simulink model "FIR_Input160M_Output200M"  (R2023b)
settings: Solver=ode45  StartTime=0.0  StopTime=100000/200e6  RelTol=1e-3  EnableMultiTasking=on
undefined symbols (not defined in the file): xc7vx485tffg1157
libraries: hdlBasic x10, aieUtilities x4, dspsrcs4 x2, hdlDSPIP x1, vmcUtilities x1
settings Model: Creator=danielm  LastModifiedBy=sdegala
settings SolverCC: AlgebraicLoopSolver=TrustRegion
settings DataIOCC: LimitDataPoints=on  SaveFormat=Array  ReturnWorkspaceOutputs=off
settings OptimizationCC: LifeSpan=inf
settings DebuggingCC: UnderspecifiedInitializationDetection=Classic  MergeDetectMultiDrivingBlocksExec=none  SolverPrmCheckMsg=warning  UnconnectedInputMsg=warning  UnconnectedOutputMsg=warning  UnconnectedLineMsg=warning  AllowSymbolicDim=off  SFUnexpectedBacktrackingDiag=warning  SFNoUnconditionalDefaultTransitionDiag=warning  SFExecutionAtInitializationDiag=none  ArithmeticOperatorsInVariantConditions=warning
settings HardwareCC: ProdBitPerPointer=32  ProdBitPerSizeT=32  ProdBitPerPtrDiffT=32  ProdLargestAtomicFloat=None  ProdIntDivRoundTo=Undefined  ProdEndianess=Unspecified  ProdWordSize=32  ProdHWDeviceType=32-bit Generic
settings ModelReferenceCC: EnableRefExpFcnMdlSchedulingChecks=on  PropagateSignalLabelsOutOfModel=off
settings SFSimCC: SimUseLocalCustomCode=off  CustomCodeUndefinedFunction=UseInterfaceOnly
settings RTWCC: RTWUseLocalCustomCode=off  DLArmComputeVersion=19.05
settings CodeAppCC: StateflowObjectComments=on
settings GRTTargetCC: TargetLangStandard=C89/C90 (ANSI)
settings ConfigComp: CovMetricSettings=dw  CovSaveCumulativeToWorkspaceVar=on  CovSaveSingleToWorkspaceVar=on  CovExternalEMLEnable=off  CovSFcnEnable=off

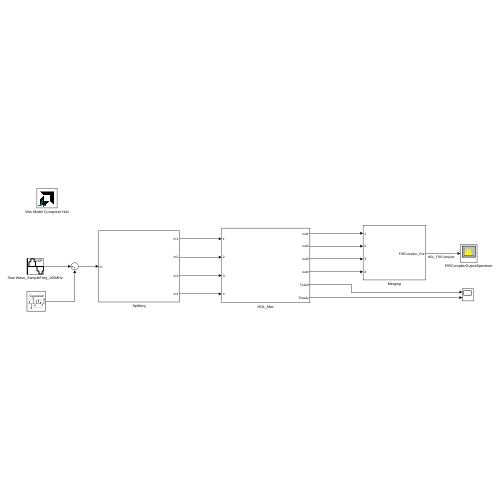
[thumbnail: Simulink's stored preview of the top-level diagram]
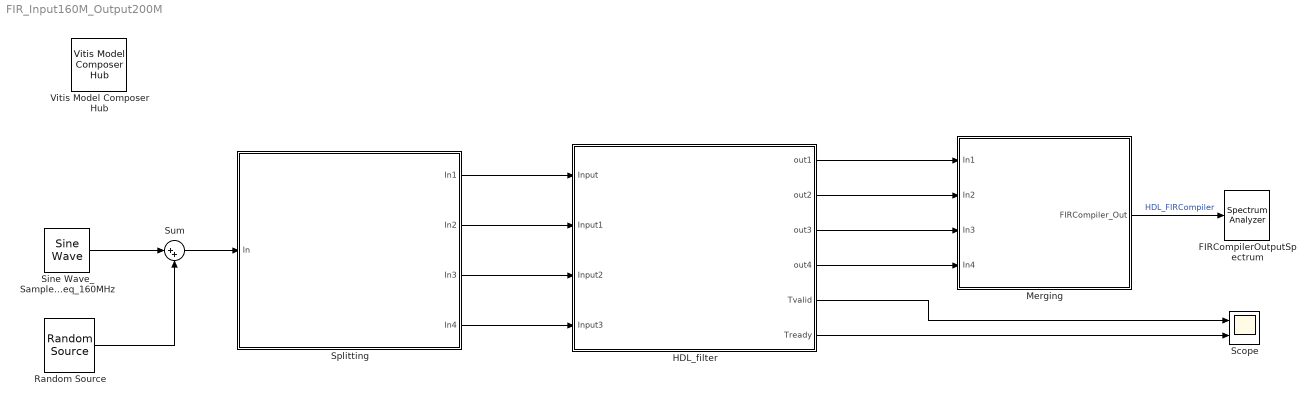
== system FIR_Input160M_Output200M ==
  FIRCompilerOutputSpectrum : SpectrumAnalyzer  WindowPosition=[1.000000,1.000000,1280.000000,744.000000,]  Visible=on  ScopeFrameLocation=window  Method=Welch  SampleRate=20000000  FrequencySpan=Span and center frequency  Span=35000000  AveragingMethod=Exponential  YLimits=[-62.95839478,117.78609735]  ShowLegend=on  ChannelNames="[\"\"]"  SelectedToolstripTab=spectrumAnalyzerToolstrip.measurementsTab  DefaultConfigurationName=spbscopes.SpectrumAnalyzerBlockCfg
  HDL_filter : Subsystem
  Merging : Subsystem
  Random Source : dspsrcs4/Random Source  SampMode=Discrete  SrcType=Gaussian  MinVal=0  MaxVal=1  MeanVal=0  VarVal=1e-5  RepMode=Specify seed  rawSeed=1  IsInherit=off  SampTime=1/160e6  SampFrame=1  OutComplex=Real  DataType=double
  Scope : Scope  NumInputPorts=2
  Sine Wave_SampleFreq_160MHz : dspsrcs4/Sine Wave  Amplitude=1  Frequency=1e6  Phase=0  SampleMode=Discrete  OutComplex=Real  CompMethod=Trigonometric fcn  TableSize=Speed  SampleTime=1/160e6  SamplesPerFrame=4  ResetState=Restart at time zero  OutputFrames=off  dataType=double  wordLen=16  udDataType=sfix(16)  fracBitsMode=Best precision  numFracBits=15  OutDataTypeStr=double  LastOutDataTypeStr=double
  Splitting : Subsystem
  Sum : Sum  Inputs=|++
  Vitis Model Composer Hub : vmcUtilities/Vitis Model Composer Hub  Tag=genX  CodeGeneration=off  SubsystemName=HDL_filter  StartColumn=1  NumberOfColumns=1  TargetDirectory=./code  exportDesign=off  analyzeDesign=off  validateDesignOnHw=off  ExportType=AI Engines  IpVendor=xilinx.com  IpLibrary=hls  IpVersion=1.0  IpHWLanguage=Verilog  AieCompilerOptions={}  AieSimulatorOptions={}  CreateTestbench=off  TestbenchStackSize=10  RunRtlSim=off  RunCSim=off  RunAieSim=off  AieSimTimeout=50000  RunAieSimProfiling=off  LaunchVitisAnalyzer=off  PlotOutput=off  RunX86Sim=off  X86SimTimeout=10  GenHwImage=off  GenLibadfXo=on  GenHwValidationCode=off  PlatformType=Not Specified  HwSystemType=Baremetal  HwValidationTarget=hw  ProjDevice=xc7vx485tffg1157-3  ProjDevicePart=xc7vx485tffg1157-3  SamplePeriod=-1  ClockFrequency=200  DataPathParallelism=1  xilinxfamily=virtex7  part=xc7vx485t  speed=-3  package=ffg1157  directory=./netlist/ip/HDL_filter/src  testbench=off  incr_netlist=off  synthesis_tool=Vivado  clock_wrapper=Clock Enables  dbl_ovrd=According to Block Masks  dcm_input_clock_period=10  sysclk_period=5  simulink_period=1/200e6  eval_field=0  LogFileName=''  NThreads=4
  wires:
  HDL_filter/5(Tvalid) -> Scope/1
  HDL_filter/6(Tready) -> Scope/2
  Splitting/1(In1) -> HDL_filter/1(Input)
  Splitting/2(In2) -> HDL_filter/2(Input1)
  Splitting/3(In3) -> HDL_filter/3(Input2)
  Splitting/4(In4) -> HDL_filter/4(Input3)
  HDL_filter/1(out1) -> Merging/1(In1)
  HDL_filter/2(out2) -> Merging/2(In2)
  HDL_filter/3(out3) -> Merging/3(In3)
  HDL_filter/4(out4) -> Merging/4(In4)
  Merging/1(FIRCompiler_Out) -> FIRCompilerOutputSpectrum/1  "HDL_FIRCompiler"
  Sine Wave_SampleFreq_160MHz/1 -> Sum/1
  Sum/1 -> Splitting/1(In)
  Random Source/1 -> Sum/2

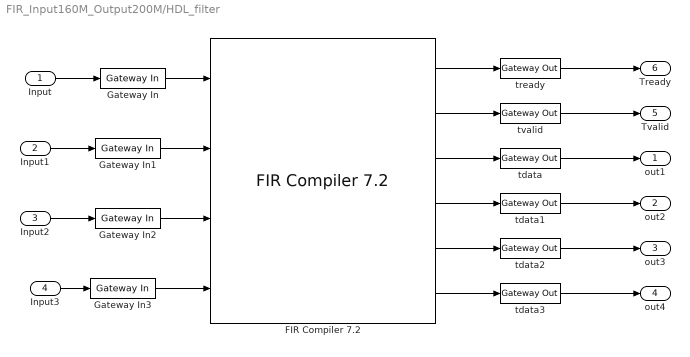
== system FIR_Input160M_Output200M/HDL_filter ==
  Input : Inport
  Input1 : Inport  Port=2
  Input2 : Inport  Port=3
  Input3 : Inport  Port=4
  FIR Compiler 7.2 : hdlDSPIP/FIR Compiler 7.2   coefficientvector=[3,2,0,-5,-14,-29,-50,-79,-115,-158,-205,-253,-296,-331,-350,-350,-326,-276,-200,-103,9,126,236,327,385,399,364,276,140,-34,-229,-424,-593,-710,-750,-694,-528,-248,139,617,1160,1732,2295,2808,3232,3535,3692,3692,3535,3232,2808,2295,1732,1160,617,139,-248,-528,-694,-750,-710,-593,-424,-229,-34,140,276,364,399,385,327,236,126,9,-103,-200,-276,-326,-350,-350,-331,-296,-253,-205,-158,-115,-79,-50,-29,-14,-5,0,2,3]  coefficient_sets=1  coefficient_reload=off  filter_type=Interpolation  rate_change_type=Fixed_Fractional  interpolation_rate=5  decimation_rate=4  zero_pack_factor=1  channel_sequence=Basic  number_channels=1  pattern_list='P4-0,P4-1,P4-2,P4-3,P4-4'  number_paths=4  ratespecification=Hardware_Oversampling_Rate  sampleperiod=5  hardwareoversamplingrate=2  coefficient_sign=Signed  quantization=Integer_Coefficients  coefficient_width=16  bestprecision=off  coefficient_fractional_bits=0  coefficient_structure=Non_Symmetric  output_rounding_mode=Full_Precision  output_width=30  filter_architecture=Systolic_Multiply_Accumulate  optimization_goal=Area  optimization_list='None'  data_buffer_type=Automatic  coefficient_buffer_type=Automatic  input_buffer_type=Automatic  output_buffer_type=Automatic  preference_for_other_storage=Automatic  multi_column_support=Automatic  columnconfig='7'  inter_column_pipe_length=4  data_has_tlast=Not_Required  m_data_has_tready=off  s_data_has_fifo=on  s_data_has_tuser=Not_Required  m_data_has_tuser=Not_Required  s_config_sync_mode=On_Vector  s_config_method=Single  num_reload_slots=1  has_aclken=off  has_aresetn=off  reset_data_vector=on  trim_axipin_name=on  simulation_type=hybrid_sim  simulation_model=sysgen:xfirv7_2_cmodel  data_path_portlist={ 's_axis_data_tdata', 'm_axis_data_tdata' }  passband_min=0.0  passband_max=0.5  stopband_min=0.5  stopband_max=1.0  filter_selection=1  gui_behaviour='Sysgen_GUI'  data_sign=Signed  data_width=16  data_fractional_bits=0  data_tuser_width=1  wrapper_available=true  ip_wrap_arbitrary_binary_point=true  ip_name=FIR Compiler  ip_version=7.2  dsptool_ready=true  ipcore_usecache=true  ipcore_useipmodelcache=true  port_translation_map={ 'aclken' => 'en', 'aresetn' => 'rst' }  run_core_at_system_period=true  ipcore_xco_need_fpga_part=true  ipcore_fpga_part=[]  XmcBlockStatus=1  maskContainerNames=tabcontainer1  block_type=fir_compiler_v7_2  block_config=sysgen:rodinimport_config  block_width=820  block_height=600
  Gateway In{,1..3} (4 alike) : hdlBasic/Gateway In  gui_display_data_type=Fixed-point  arith_type=Signed (2's comp)  n_bits=16  bin_pt=14  preci_type=Single  exp_width=8  frac_width=24  rows=1  columns=1  quantization="Round  (unbiased: +/- Inf)"  overflow=Saturate  period=1/40e6  UseAsADC=off  ADCChannel='1'  interface=None  automatic_assignment=on  address_offset=hex2dec('00')  intf_name=''  intf_description=''  default_value=0  timing_constraint=None  locs_specified=off  LOCs={}  io_standard={}  inherit_from_input=off  hdl_port=on  XmcBlockStatus=1  maskContainerNames=group4  block_type=gatewayin  block_config=sysgen:gateway_in_config  block_width_w=590  block_height_w=620  block_width=640  block_height=850
  tdata{,1..3} (4 alike) : hdlBasic/Gateway Out  inherit_from_input=off  hdl_port=on  rows=1  columns=1  UseAsDAC=off  DACChannel='1'  interface=None  automatic_assignment=on  address_offset=hex2dec('00')  intf_name=''  intf_description=''  timing_constraint=None  locs_specified=off  LOCs={}  io_standard={}  XmcBlockStatus=1  maskContainerNames=group4  block_type=gatewayout  block_config=sysgen:gateway_out_config  block_width_w=590  block_height_w=620  block_width=620  block_height=750
  tready : hdlBasic/Gateway Out  inherit_from_input=off  hdl_port=on  rows=1  columns=1  UseAsDAC=off  DACChannel='1'  interface=None  automatic_assignment=on  address_offset=hex2dec('00')  intf_name=''  intf_description=''  timing_constraint=None  locs_specified=off  LOCs={}  io_standard={}  XmcBlockStatus=1  maskContainerNames=group4  block_type=gatewayout  block_config=sysgen:gateway_out_config  block_width_w=590  block_height_w=620  block_width=620  block_height=750
  tvalid : hdlBasic/Gateway Out  inherit_from_input=off  hdl_port=on  rows=1  columns=1  UseAsDAC=off  DACChannel='1'  interface=None  automatic_assignment=on  address_offset=hex2dec('00')  intf_name=''  intf_description=''  timing_constraint=None  locs_specified=off  LOCs={}  io_standard={}  XmcBlockStatus=1  maskContainerNames=group4  block_type=gatewayout  block_config=sysgen:gateway_out_config  block_width_w=590  block_height_w=620  block_width=620  block_height=750
  out1 : Outport
  out2 : Outport  Port=2
  out3 : Outport  Port=3
  out4 : Outport  Port=4
  Tvalid : Outport  Port=5
  Tready : Outport  Port=6
  wires:
  Gateway In/1 -> FIR Compiler 7.2/1
  Input/1 -> Gateway In/1
  FIR Compiler 7.2/3 -> tdata/1
  FIR Compiler 7.2/2 -> tvalid/1
  FIR Compiler 7.2/1 -> tready/1
  tdata/1 -> out1/1
  tvalid/1 -> Tvalid/1
  tready/1 -> Tready/1
  Input1/1 -> Gateway In1/1
  Gateway In1/1 -> FIR Compiler 7.2/2
  Input2/1 -> Gateway In2/1
  Gateway In2/1 -> FIR Compiler 7.2/3
  Gateway In3/1 -> FIR Compiler 7.2/4
  Input3/1 -> Gateway In3/1
  FIR Compiler 7.2/4 -> tdata1/1
  tdata1/1 -> out2/1
  FIR Compiler 7.2/5 -> tdata2/1
  tdata2/1 -> out3/1
  FIR Compiler 7.2/6 -> tdata3/1
  tdata3/1 -> out4/1

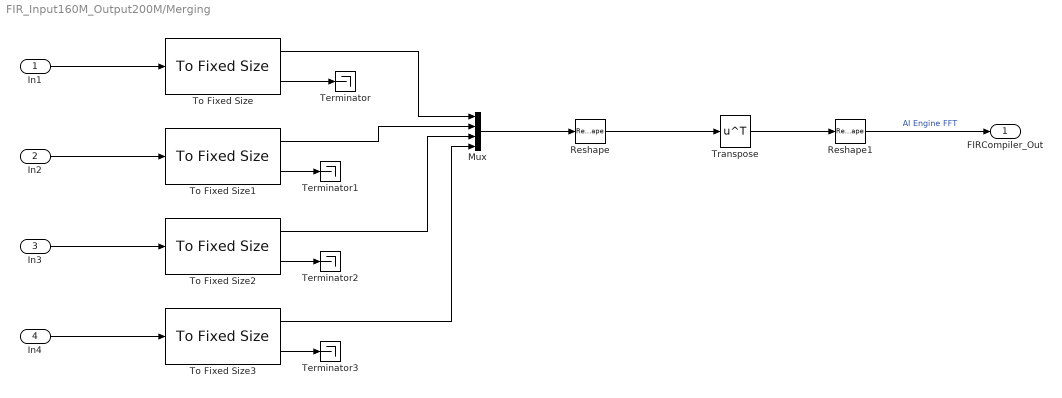
== system FIR_Input160M_Output200M/Merging ==
  In1 : Inport
  In2 : Inport  Port=2
  In3 : Inport  Port=3
  In4 : Inport  Port=4
  Mux : Mux
  Reshape : Reshape  OutputDimensionality=Customize  OutputDimensions=[1, 4]
  Reshape1 : Reshape  OutputDimensions=[1, 10]
  Terminator{,1..3} (4 alike) : Terminator
  To Fixed Size{,1..3} (4 alike) : aieUtilities/To Fixed Size  Mode=Produce a valid output signal  OutputSize=Inherit: Same as input  CopyMethod=Buffer samples to form output  HasStatusOutput=on
  Transpose : Math  Operator=transpose
  FIRCompiler_Out : Outport
  wires:
  Reshape/1 -> Transpose/1
  To Fixed Size1/2 -> Terminator1/1
  To Fixed Size1/1 -> Mux/2
  In2/1 -> To Fixed Size1/1
  To Fixed Size/2 -> Terminator/1
  Transpose/1 -> Reshape1/1
  To Fixed Size/1 -> Mux/1
  Mux/1 -> Reshape/1
  Reshape1/1 -> FIRCompiler_Out/1  "AI Engine FFT"
  In1/1 -> To Fixed Size/1
  To Fixed Size2/2 -> Terminator2/1
  In4/1 -> To Fixed Size3/1
  To Fixed Size3/1 -> Mux/4
  To Fixed Size3/2 -> Terminator3/1
  In3/1 -> To Fixed Size2/1
  To Fixed Size2/1 -> Mux/3

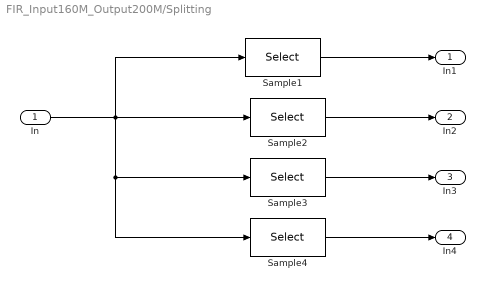
== system FIR_Input160M_Output200M/Splitting ==
  In : Inport
  Sample1 : Selector  InputPortWidth=4  IndexOptions=Index vector (dialog)  Indices=1:4:4  OutputSizes=1
  Sample2 : Selector  InputPortWidth=4  IndexOptions=Index vector (dialog)  Indices=2:4:4  OutputSizes=1
  Sample3 : Selector  InputPortWidth=4  IndexOptions=Index vector (dialog)  Indices=3:4:4  OutputSizes=1
  Sample4 : Selector  InputPortWidth=4  IndexOptions=Index vector (dialog)  Indices=4:4:4  OutputSizes=1
  In1 : Outport
  In2 : Outport  Port=2
  In3 : Outport  Port=3
  In4 : Outport  Port=4
  wires:
  In/1 -> Sample4/1, Sample3/1, Sample2/1, Sample1/1
  Sample2/1 -> In2/1
  Sample1/1 -> In1/1
  Sample3/1 -> In3/1
  Sample4/1 -> In4/1
